simulink subsystem "PvtSubSys_DMS"  (R2020b)
settings: Solver=VariableStepAuto  StartTime=0.0  StopTime=10.0  RelTol=1e-3
undefined symbols (not defined in the file): DMS5, DS, P_DMS_tDSGoodUnbeliv2LowDistrctn, P_DMS_tDSGoodUnbeliv2LowDrowsns, P_DMS_tDSGoodUnbeliv2MidDistractn, P_DMS_tDSGoodUnbeliv2MidDrowsns, P_DMS_tDSLow2MidDistractn, P_DMS_tDSLow2MidDrowsns, P_DMS_tDSOther2Hi1Distractn, P_DMS_tDSOther2Hi1Drowsns, P_DMS_tDSOther2Hi2Distractn, P_DMS_tDSOther2Hi2Drowsns
libraries: simulink x92, TrueDurationTime x22
(part 1 of 2)
settings Model: Creator=GW00184765  LastModifiedBy=GW00133806

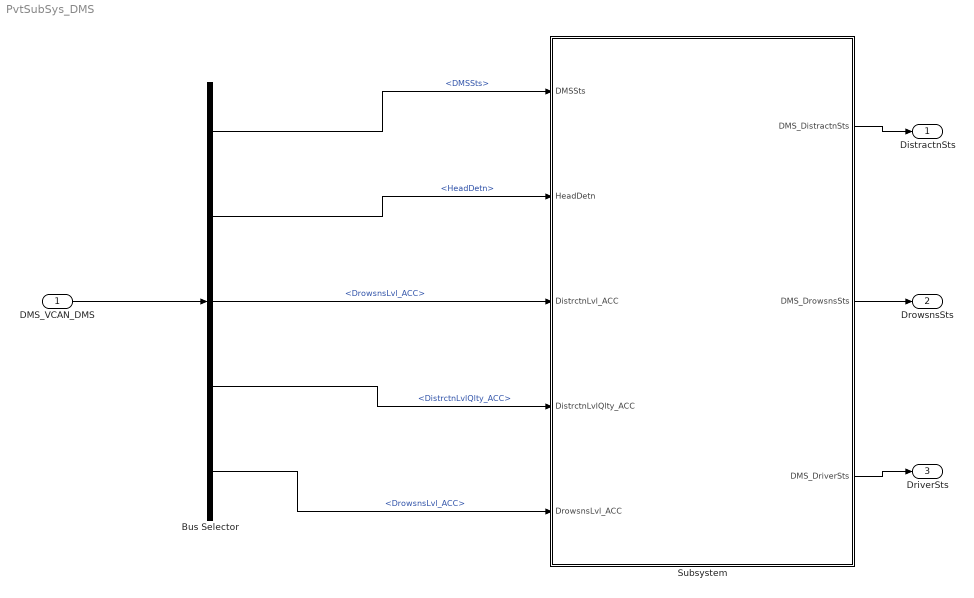
== system PvtSubSys_DMS ==
  DMS_VCAN_DMS : Inport  OutDataTypeStr=Bus: VCAN_DMS_MSG_BUS  PortDimensions=1  BusOutputAsStruct=on
  Bus Selector : BusSelector  OutputSignals=DMSSts,HeadDetn,DrowsnsLvl_ACC,DistrctnLvlQlty_ACC,DrowsnsLvl_ACC
  Subsystem : Subsystem
  DistractnSts : Outport  OutDataTypeStr=uint8  PortDimensions=1  BusOutputAsStruct=on
  DrowsnsSts : Outport  Port=2  OutDataTypeStr=uint8  PortDimensions=1  BusOutputAsStruct=on
  DriverSts : Outport  Port=3  OutDataTypeStr=uint8  PortDimensions=1  BusOutputAsStruct=on
  wires:
  Bus Selector/5 -> Subsystem/5(DrowsnsLvl_ACC)  "<DrowsnsLvl_ACC>"
  Bus Selector/2 -> Subsystem/2(HeadDetn)  "<HeadDetn>"
  Bus Selector/4 -> Subsystem/4(DistrctnLvlQlty_ACC)  "<DistrctnLvlQlty_ACC>"
  DMS_VCAN_DMS/1 -> Bus Selector/1
  Bus Selector/1 -> Subsystem/1(DMSSts)  "<DMSSts>"
  Bus Selector/3 -> Subsystem/3(DistrctnLvl_ACC)  "<DrowsnsLvl_ACC>"
  Subsystem/2(DMS_DrowsnsSts) -> DrowsnsSts/1
  Subsystem/1(DMS_DistractnSts) -> DistractnSts/1
  Subsystem/3(DMS_DriverSts) -> DriverSts/1

== system PvtSubSys_DMS/Subsystem ==
  DMSSts : Inport  OutDataTypeStr=uint8  PortDimensions=1  Interpolate=off  BusOutputAsStruct=on
  HeadDetn : Inport  Port=2  OutDataTypeStr=boolean  PortDimensions=1  Interpolate=off  BusOutputAsStruct=on
  DistrctnLvl_ACC : Inport  Port=3  OutDataTypeStr=uint8  PortDimensions=1  Interpolate=off  BusOutputAsStruct=on
  DistrctnLvlQlty_ACC : Inport  Port=4  OutDataTypeStr=uint8  PortDimensions=1  Interpolate=off  BusOutputAsStruct=on
  DrowsnsLvl_ACC : Inport  Port=5  OutDataTypeStr=uint8  PortDimensions=1  Interpolate=off  BusOutputAsStruct=on
  DS : Subsystem  AncestorBlock=DMS5/DS
  DMS_DistractnSts : Outport
  DMS_DrowsnsSts : Outport  Port=2
  DMS_DriverSts : Outport  Port=3
  wires:
  DrowsnsLvl_ACC/1 -> DS/5(canDrowsnsLevel)
  DistrctnLvlQlty_ACC/1 -> DS/4(canDistrctnQlty)
  DistrctnLvl_ACC/1 -> DS/3(canDistrctnLevel)
  DMSSts/1 -> DS/1(canDMSSts)
  HeadDetn/1 -> DS/2(canHeadDetn)
  DS/3(DriverSts) -> DMS_DriverSts/1  "DMS_DriverSts"
  DS/2(DrowsnsSts) -> DMS_DrowsnsSts/1  "DMS_DrowsnsSts"
  DS/1(DistractnSts) -> DMS_DistractnSts/1  "DMS_DistractnSts"

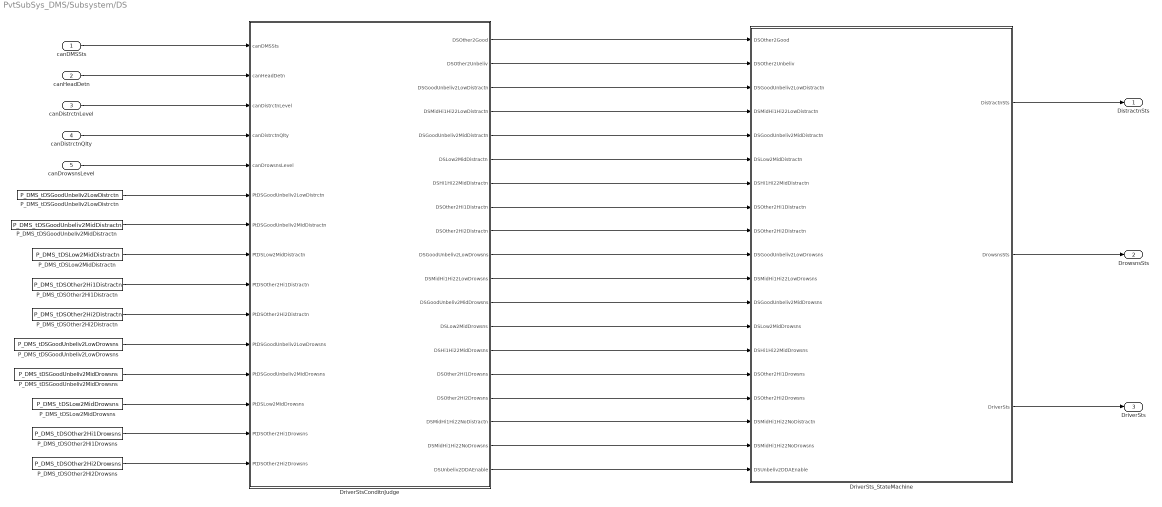
== system PvtSubSys_DMS/Subsystem/DS ==
  canDMSSts : Inport  OutDataTypeStr=uint8
  canHeadDetn : Inport  Port=2  OutDataTypeStr=boolean
  canDistrctnLevel : Inport  Port=3  OutDataTypeStr=uint8
  canDistrctnQlty : Inport  Port=4  OutDataTypeStr=uint8
  canDrowsnsLevel : Inport  Port=5  OutDataTypeStr=uint8
  DriverStsConditnJudge : Subsystem
  DriverSts_StateMachine : Stateflow chart  TreatAsAtomicUnit=on
  P_DMS_tDSGoodUnbeliv2LowDistrctn : Constant  Value=P_DMS_tDSGoodUnbeliv2LowDistrctn
  P_DMS_tDSGoodUnbeliv2LowDrowsns : Constant  Value=P_DMS_tDSGoodUnbeliv2LowDrowsns
  P_DMS_tDSGoodUnbeliv2MidDistractn : Constant  Value=P_DMS_tDSGoodUnbeliv2MidDistractn
  P_DMS_tDSGoodUnbeliv2MidDrowsns : Constant  Value=P_DMS_tDSGoodUnbeliv2MidDrowsns
  P_DMS_tDSLow2MidDistractn : Constant  Value=P_DMS_tDSLow2MidDistractn
  P_DMS_tDSLow2MidDrowsns : Constant  Value=P_DMS_tDSLow2MidDrowsns
  P_DMS_tDSOther2Hi1Distractn : Constant  Value=P_DMS_tDSOther2Hi1Distractn
  P_DMS_tDSOther2Hi1Drowsns : Constant  Value=P_DMS_tDSOther2Hi1Drowsns
  P_DMS_tDSOther2Hi2Distractn : Constant  Value=P_DMS_tDSOther2Hi2Distractn
  P_DMS_tDSOther2Hi2Drowsns : Constant  Value=P_DMS_tDSOther2Hi2Drowsns
  DistractnSts : Outport  OutDataTypeStr=uint8
  DrowsnsSts : Outport  Port=2  OutDataTypeStr=uint8
  DriverSts : Outport  Port=3  OutDataTypeStr=uint8
  wires:
  canDistrctnLevel/1 -> DriverStsConditnJudge/3(canDistrctnLevel)
  canDistrctnQlty/1 -> DriverStsConditnJudge/4(canDistrctnQlty)
  canHeadDetn/1 -> DriverStsConditnJudge/2(canHeadDetn)
  canDrowsnsLevel/1 -> DriverStsConditnJudge/5(canDrowsnsLevel)
  canDMSSts/1 -> DriverStsConditnJudge/1(canDMSSts)
  P_DMS_tDSGoodUnbeliv2LowDistrctn/1 -> DriverStsConditnJudge/6(PtDSGoodUnbeliv2LowDistrctn)
  P_DMS_tDSGoodUnbeliv2MidDistractn/1 -> DriverStsConditnJudge/7(PtDSGoodUnbeliv2MidDistractn)
  P_DMS_tDSLow2MidDistractn/1 -> DriverStsConditnJudge/8(PtDSLow2MidDistractn)
  P_DMS_tDSOther2Hi1Distractn/1 -> DriverStsConditnJudge/9(PtDSOther2Hi1Distractn)
  P_DMS_tDSOther2Hi2Distractn/1 -> DriverStsConditnJudge/10(PtDSOther2Hi2Distractn)
  P_DMS_tDSGoodUnbeliv2LowDrowsns/1 -> DriverStsConditnJudge/11(PtDSGoodUnbeliv2LowDrowsns)
  P_DMS_tDSGoodUnbeliv2MidDrowsns/1 -> DriverStsConditnJudge/12(PtDSGoodUnbeliv2MidDrowsns)
  P_DMS_tDSLow2MidDrowsns/1 -> DriverStsConditnJudge/13(PtDSLow2MidDrowsns)
  P_DMS_tDSOther2Hi1Drowsns/1 -> DriverStsConditnJudge/14(PtDSOther2Hi1Drowsns)
  P_DMS_tDSOther2Hi2Drowsns/1 -> DriverStsConditnJudge/15(PtDSOther2Hi2Drowsns)
  DriverStsConditnJudge/1(DSOther2Good) -> DriverSts_StateMachine/1(DSOther2Good)
  DriverStsConditnJudge/2(DSOther2Unbeliv) -> DriverSts_StateMachine/2(DSOther2Unbeliv)
  DriverStsConditnJudge/3(DSGoodUnbeliv2LowDistractn) -> DriverSts_StateMachine/3(DSGoodUnbeliv2LowDistractn)
  DriverStsConditnJudge/4(DSMidHi1Hi22LowDistractn) -> DriverSts_StateMachine/4(DSMidHi1Hi22LowDistractn)
  DriverStsConditnJudge/5(DSGoodUnbeliv2MidDistractn) -> DriverSts_StateMachine/5(DSGoodUnbeliv2MidDistractn)
  DriverStsConditnJudge/6(DSLow2MidDistractn) -> DriverSts_StateMachine/6(DSLow2MidDistractn)
  DriverStsConditnJudge/7(DSHi1Hi22MidDistractn) -> DriverSts_StateMachine/7(DSHi1Hi22MidDistractn)
  DriverStsConditnJudge/8(DSOther2Hi1Distractn) -> DriverSts_StateMachine/8(DSOther2Hi1Distractn)
  DriverStsConditnJudge/9(DSOther2Hi2Distractn) -> DriverSts_StateMachine/9(DSOther2Hi2Distractn)
  DriverStsConditnJudge/10(DSGoodUnbeliv2LowDrowsns) -> DriverSts_StateMachine/10(DSGoodUnbeliv2LowDrowsns)
  DriverStsConditnJudge/11(DSMidHi1Hi22LowDrowsns) -> DriverSts_StateMachine/11(DSMidHi1Hi22LowDrowsns)
  DriverStsConditnJudge/12(DSGoodUnbeliv2MidDrowsns) -> DriverSts_StateMachine/12(DSGoodUnbeliv2MidDrowsns)
  DriverStsConditnJudge/13(DSLow2MidDrowsns) -> DriverSts_StateMachine/13(DSLow2MidDrowsns)
  DriverStsConditnJudge/14(DSHi1Hi22MidDrowsns) -> DriverSts_StateMachine/14(DSHi1Hi22MidDrowsns)
  DriverStsConditnJudge/15(DSOther2Hi1Drowsns) -> DriverSts_StateMachine/15(DSOther2Hi1Drowsns)
  DriverStsConditnJudge/16(DSOther2Hi2Drowsns) -> DriverSts_StateMachine/16(DSOther2Hi2Drowsns)
  DriverStsConditnJudge/17(DSMidHi1Hi22NoDistractn) -> DriverSts_StateMachine/17(DSMidHi1Hi22NoDistractn)
  DriverStsConditnJudge/18(DSMidHi1Hi22NoDrowsns) -> DriverSts_StateMachine/18(DSMidHi1Hi22NoDrowsns)
  DriverStsConditnJudge/19(DSUnbeliv2DDAEnable) -> DriverSts_StateMachine/19(DSUnbeliv2DDAEnable)
  DriverSts_StateMachine/1(DistractnSts) -> DistractnSts/1
  DriverSts_StateMachine/2(DrowsnsSts) -> DrowsnsSts/1
  DriverSts_StateMachine/3(DriverSts) -> DriverSts/1

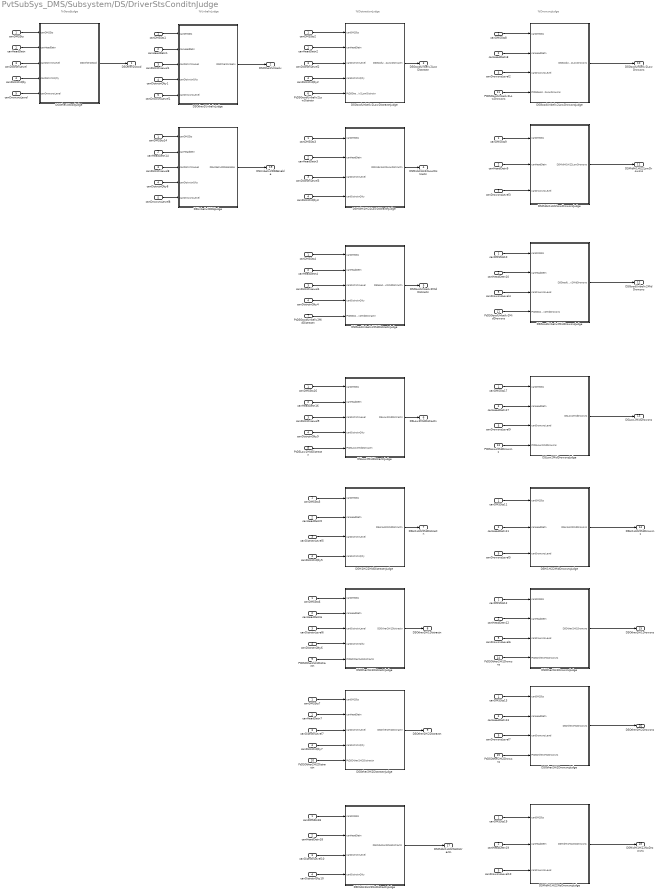
== system PvtSubSys_DMS/Subsystem/DS/DriverStsConditnJudge ==
  note: %GoodJudge
  note: %UnbelivJudge
  note: %DistractionJudge
  note: %DrowsnsJudge
  canDMSSts : Inport
  canHeadDetn : Inport  Port=2
  canDistrctnLevel : Inport  Port=3
  canDistrctnQlty : Inport  Port=4
  canDrowsnsLevel : Inport  Port=5
  PtDSGoodUnbeliv2LowDistrctn : Inport  Port=6
  PtDSGoodUnbeliv2MidDistractn : Inport  Port=7
  PtDSLow2MidDistractn : Inport  Port=8
  PtDSOther2Hi1Distractn : Inport  Port=9
  PtDSOther2Hi2Distractn : Inport  Port=10
  PtDSGoodUnbeliv2LowDrowsns : Inport  Port=11
  PtDSGoodUnbeliv2MidDrowsns : Inport  Port=12
  PtDSLow2MidDrowsns : Inport  Port=13
  PtDSOther2Hi1Drowsns : Inport  Port=14
  PtDSOther2Hi2Drowsns : Inport  Port=15
  DSGoodUnbeliv2LowDistractnJudge : Subsystem
  DSGoodUnbeliv2LowDrowsnsJudge : Subsystem
  DSGoodUnbeliv2MidDistractnJudge : Subsystem
  DSGoodUnbeliv2MidDrowsnsJudge : Subsystem
  DSHi1Hi22MidDistractnJudge : Subsystem
  DSHi1Hi22MidDrowsnsJudge : Subsystem
  DSLow2MidDistractnJudge : Subsystem
  DSLow2MidDrowsnsJudge : Subsystem
  DSMidHi1Hi22LowDistractnJudge : Subsystem
  DSMidHi1Hi22LowDrowsnsJudge : Subsystem
  DSMidHi1Hi22NoDistractnJudge : Subsystem
  DSMidHi1Hi22NoDrowsnsJudge : Subsystem
  DSOther2GoodJudge : Subsystem
  DSOther2Hi1DistractnJudge : Subsystem
  DSOther2Hi1DrowsnsJudge : Subsystem
  DSOther2Hi2DistractnJudge : Subsystem
  DSOther2Hi2DrowsnsJudge : Subsystem
  DSOther2UnbelivJudge : Subsystem
  DSUnbeliv2DDAJudge : Subsystem
  canDMSSts{1..14,16..19} (18 alike) : InportShadow
  canDistrctnLevel{1..10} (10 alike) : InportShadow  Port=3
  canDistrctnQlty{1..10} (10 alike) : InportShadow  Port=4
  canDrowsnsLevel{1..10} (10 alike) : InportShadow  Port=5
  canHeadDetn{1..14,16..19} (18 alike) : InportShadow  Port=2
  DSOther2Good : Outport
  DSOther2Unbeliv : Outport  Port=2
  DSGoodUnbeliv2LowDistractn : Outport  Port=3
  DSMidHi1Hi22LowDistractn : Outport  Port=4
  DSGoodUnbeliv2MidDistractn : Outport  Port=5
  DSLow2MidDistractn : Outport  Port=6
  DSHi1Hi22MidDistractn : Outport  Port=7
  DSOther2Hi1Distractn : Outport  Port=8
  DSOther2Hi2Distractn : Outport  Port=9
  DSGoodUnbeliv2LowDrowsns : Outport  Port=10
  DSMidHi1Hi22LowDrowsns : Outport  Port=11
  DSGoodUnbeliv2MidDrowsns : Outport  Port=12
  DSLow2MidDrowsns : Outport  Port=13
  DSHi1Hi22MidDrowsns : Outport  Port=14
  DSOther2Hi1Drowsns : Outport  Port=15
  DSOther2Hi2Drowsns : Outport  Port=16
  DSMidHi1Hi22NoDistractn : Outport  Port=17
  DSMidHi1Hi22NoDrowsns : Outport  Port=18
  DSUnbeliv2DDAEnable : Outport  Port=19
  wires:
  canDMSSts/1 -> DSOther2GoodJudge/1(canDMSSts)
  DSOther2GoodJudge/1(DSOther2Good) -> DSOther2Good/1
  canHeadDetn/1 -> DSOther2GoodJudge/2(canHeadDetn)
  canDistrctnLevel/1 -> DSOther2GoodJudge/3(canDistrctnLevel)
  canDistrctnQlty/1 -> DSOther2GoodJudge/4(canDistrctnQlty)
  canDrowsnsLevel/1 -> DSOther2GoodJudge/5(canDrowsnsLevel)
  canDMSSts1/1 -> DSOther2UnbelivJudge/1(canDMSSts)
  canHeadDetn1/1 -> DSOther2UnbelivJudge/2(canHeadDetn)
  canDistrctnLevel1/1 -> DSOther2UnbelivJudge/3(canDistrctnLevel)
  canDistrctnQlty1/1 -> DSOther2UnbelivJudge/4(canDistrctnQlty)
  canDrowsnsLevel1/1 -> DSOther2UnbelivJudge/5(canDrowsnsLevel)
  DSOther2UnbelivJudge/1(DSOther2Unbeliv) -> DSOther2Unbeliv/1
  DSGoodUnbeliv2LowDistractnJudge/1(DSGoodUnbeliv2LowDistractn) -> DSGoodUnbeliv2LowDistractn/1
  canDMSSts2/1 -> DSGoodUnbeliv2LowDistractnJudge/1(canDMSSts)
  canHeadDetn2/1 -> DSGoodUnbeliv2LowDistractnJudge/2(canHeadDetn)
  canDistrctnLevel2/1 -> DSGoodUnbeliv2LowDistractnJudge/3(canDistrctnLevel)
  canDistrctnQlty2/1 -> DSGoodUnbeliv2LowDistractnJudge/4(canDistrctnQlty)
  canDMSSts3/1 -> DSMidHi1Hi22LowDistractnJudge/1(canDMSSts)
  canHeadDetn3/1 -> DSMidHi1Hi22LowDistractnJudge/2(canHeadDetn)
  canDistrctnLevel3/1 -> DSMidHi1Hi22LowDistractnJudge/3(canDistrctnLevel)
  canDistrctnQlty3/1 -> DSMidHi1Hi22LowDistractnJudge/4(canDistrctnQlty)
  DSMidHi1Hi22LowDistractnJudge/1(DSMidHi1Hi22LowDistractn) -> DSMidHi1Hi22LowDistractn/1
  canDMSSts4/1 -> DSGoodUnbeliv2MidDistractnJudge/1(canDMSSts)
  canHeadDetn4/1 -> DSGoodUnbeliv2MidDistractnJudge/2(canHeadDetn)
  canDistrctnLevel4/1 -> DSGoodUnbeliv2MidDistractnJudge/3(canDistrctnLevel)
  canDistrctnQlty4/1 -> DSGoodUnbeliv2MidDistractnJudge/4(canDistrctnQlty)
  DSGoodUnbeliv2MidDistractnJudge/1(DSGoodUnbeliv2MidDistractn) -> DSGoodUnbeliv2MidDistractn/1
  canDMSSts5/1 -> DSHi1Hi22MidDistractnJudge/1(canDMSSts)
  canHeadDetn5/1 -> DSHi1Hi22MidDistractnJudge/2(canHeadDetn)
  canDistrctnLevel5/1 -> DSHi1Hi22MidDistractnJudge/3(canDistrctnLevel)
  canDistrctnQlty5/1 -> DSHi1Hi22MidDistractnJudge/4(canDistrctnQlty)
  DSHi1Hi22MidDistractnJudge/1(DSHi1Hi22MidDistractn) -> DSHi1Hi22MidDistractn/1
  DSOther2Hi1DistractnJudge/1(DSOther2Hi1Distractn) -> DSOther2Hi1Distractn/1
  canDMSSts6/1 -> DSOther2Hi1DistractnJudge/1(canDMSSts)
  canHeadDetn6/1 -> DSOther2Hi1DistractnJudge/2(canHeadDetn)
  canDistrctnLevel6/1 -> DSOther2Hi1DistractnJudge/3(canDistrctnLevel)
  canDistrctnQlty6/1 -> DSOther2Hi1DistractnJudge/4(canDistrctnQlty)
  DSOther2Hi2DistractnJudge/1(DSOther2Hi2Distractn) -> DSOther2Hi2Distractn/1
  canDMSSts7/1 -> DSOther2Hi2DistractnJudge/1(canDMSSts)
  canHeadDetn7/1 -> DSOther2Hi2DistractnJudge/2(canHeadDetn)
  canDistrctnLevel7/1 -> DSOther2Hi2DistractnJudge/3(canDistrctnLevel)
  canDistrctnQlty7/1 -> DSOther2Hi2DistractnJudge/4(canDistrctnQlty)
  DSGoodUnbeliv2LowDrowsnsJudge/1(DSGoodUnbeliv2LowDrowsns) -> DSGoodUnbeliv2LowDrowsns/1
  canDMSSts8/1 -> DSGoodUnbeliv2LowDrowsnsJudge/1(canDMSSts)
  canHeadDetn8/1 -> DSGoodUnbeliv2LowDrowsnsJudge/2(canHeadDetn)
  canDrowsnsLevel2/1 -> DSGoodUnbeliv2LowDrowsnsJudge/3(canDrowsnsLevel)
  DSMidHi1Hi22LowDrowsnsJudge/1(DSMidHi1Hi22LowDrowsns) -> DSMidHi1Hi22LowDrowsns/1
  canDMSSts9/1 -> DSMidHi1Hi22LowDrowsnsJudge/1(canDMSSts)
  canHeadDetn9/1 -> DSMidHi1Hi22LowDrowsnsJudge/2(canHeadDetn)
  canDrowsnsLevel3/1 -> DSMidHi1Hi22LowDrowsnsJudge/3(canDrowsnsLevel)
  canDMSSts10/1 -> DSGoodUnbeliv2MidDrowsnsJudge/1(canDMSSts)
  canHeadDetn10/1 -> DSGoodUnbeliv2MidDrowsnsJudge/2(canHeadDetn)
  canDrowsnsLevel4/1 -> DSGoodUnbeliv2MidDrowsnsJudge/3(canDrowsnsLevel)
  DSGoodUnbeliv2MidDrowsnsJudge/1(DSGoodUnbeliv2MidDrowsns) -> DSGoodUnbeliv2MidDrowsns/1
  DSHi1Hi22MidDrowsnsJudge/1(DSHi1Hi22MidDrowsns) -> DSHi1Hi22MidDrowsns/1
  canDrowsnsLevel5/1 -> DSHi1Hi22MidDrowsnsJudge/3(canDrowsnsLevel)
  canHeadDetn11/1 -> DSHi1Hi22MidDrowsnsJudge/2(canHeadDetn)
  canDMSSts11/1 -> DSHi1Hi22MidDrowsnsJudge/1(canDMSSts)
  canDMSSts12/1 -> DSOther2Hi1DrowsnsJudge/1(canDMSSts)
  canHeadDetn12/1 -> DSOther2Hi1DrowsnsJudge/2(canHeadDetn)
  canDrowsnsLevel6/1 -> DSOther2Hi1DrowsnsJudge/3(canDrowsnsLevel)
  DSOther2Hi1DrowsnsJudge/1(DSOther2Hi1Drowsns) -> DSOther2Hi1Drowsns/1
  canDrowsnsLevel7/1 -> DSOther2Hi2DrowsnsJudge/3(canDrowsnsLevel)
  canHeadDetn13/1 -> DSOther2Hi2DrowsnsJudge/2(canHeadDetn)
  canDMSSts13/1 -> DSOther2Hi2DrowsnsJudge/1(canDMSSts)
  DSOther2Hi2DrowsnsJudge/1(DSOther2Hi2Drowsns) -> DSOther2Hi2Drowsns/1
  DSLow2MidDistractnJudge/1(DSLow2MidDistractn) -> DSLow2MidDistractn/1
  canDistrctnQlty9/1 -> DSLow2MidDistractnJudge/4(canDistrctnQlty)
  canDistrctnLevel9/1 -> DSLow2MidDistractnJudge/3(canDistrctnLevel)
  canHeadDetn16/1 -> DSLow2MidDistractnJudge/2(canHeadDetn)
  canDMSSts16/1 -> DSLow2MidDistractnJudge/1(canDMSSts)
  canDrowsnsLevel9/1 -> DSLow2MidDrowsnsJudge/3(canDrowsnsLevel)
  canHeadDetn17/1 -> DSLow2MidDrowsnsJudge/2(canHeadDetn)
  canDMSSts17/1 -> DSLow2MidDrowsnsJudge/1(canDMSSts)
  DSLow2MidDrowsnsJudge/1(DSLow2MidDrowsns) -> DSLow2MidDrowsns/1
  canDistrctnQlty10/1 -> DSMidHi1Hi22NoDistractnJudge/4(canDistrctnQlty)
  canDistrctnLevel10/1 -> DSMidHi1Hi22NoDistractnJudge/3(canDistrctnLevel)
  canHeadDetn18/1 -> DSMidHi1Hi22NoDistractnJudge/2(canHeadDetn)
  canDMSSts18/1 -> DSMidHi1Hi22NoDistractnJudge/1(canDMSSts)
  DSMidHi1Hi22NoDistractnJudge/1(DSMidHi1Hi22NoDistractn) -> DSMidHi1Hi22NoDistractn/1
  canDrowsnsLevel10/1 -> DSMidHi1Hi22NoDrowsnsJudge/3(canDrowsnsLevel)
  canHeadDetn19/1 -> DSMidHi1Hi22NoDrowsnsJudge/2(canHeadDetn)
  canDMSSts19/1 -> DSMidHi1Hi22NoDrowsnsJudge/1(canDMSSts)
  DSMidHi1Hi22NoDrowsnsJudge/1(DSMidHi1Hi22NoDrowsns) -> DSMidHi1Hi22NoDrowsns/1
  canDrowsnsLevel8/1 -> DSUnbeliv2DDAJudge/5(canDrowsnsLevel)
  canDistrctnQlty8/1 -> DSUnbeliv2DDAJudge/4(canDistrctnQlty)
  canDistrctnLevel8/1 -> DSUnbeliv2DDAJudge/3(canDistrctnLevel)
  canHeadDetn14/1 -> DSUnbeliv2DDAJudge/2(canHeadDetn)
  canDMSSts14/1 -> DSUnbeliv2DDAJudge/1(canDMSSts)
  DSUnbeliv2DDAJudge/1(DSUnbeliv2DDAEnable) -> DSUnbeliv2DDAEnable/1
  PtDSGoodUnbeliv2LowDistrctn/1 -> DSGoodUnbeliv2LowDistractnJudge/5(PtDSGoodUnbeliv2LowDistrctn)
  PtDSGoodUnbeliv2MidDistractn/1 -> DSGoodUnbeliv2MidDistractnJudge/5(PtDSGoodUnbeliv2MidDistractn)
  PtDSLow2MidDistractn/1 -> DSLow2MidDistractnJudge/5(PtDSLow2MidDistractn)
  PtDSOther2Hi1Distractn/1 -> DSOther2Hi1DistractnJudge/5(PtDSOther2Hi1Distractn)
  PtDSOther2Hi2Distractn/1 -> DSOther2Hi2DistractnJudge/5(PtDSOther2Hi2Distractn)
  PtDSGoodUnbeliv2LowDrowsns/1 -> DSGoodUnbeliv2LowDrowsnsJudge/4(PtDSGoodUnbeliv2LowDrowsns)
  PtDSGoodUnbeliv2MidDrowsns/1 -> DSGoodUnbeliv2MidDrowsnsJudge/4(PtDSGoodUnbeliv2MidDrowsns)
  PtDSLow2MidDrowsns/1 -> DSLow2MidDrowsnsJudge/4(PtDSLow2MidDrowsns)
  PtDSOther2Hi1Drowsns/1 -> DSOther2Hi1DrowsnsJudge/4(PtDSOther2Hi1Drowsns)
  PtDSOther2Hi2Drowsns/1 -> DSOther2Hi2DrowsnsJudge/4(PtDSOther2Hi2Drowsns)

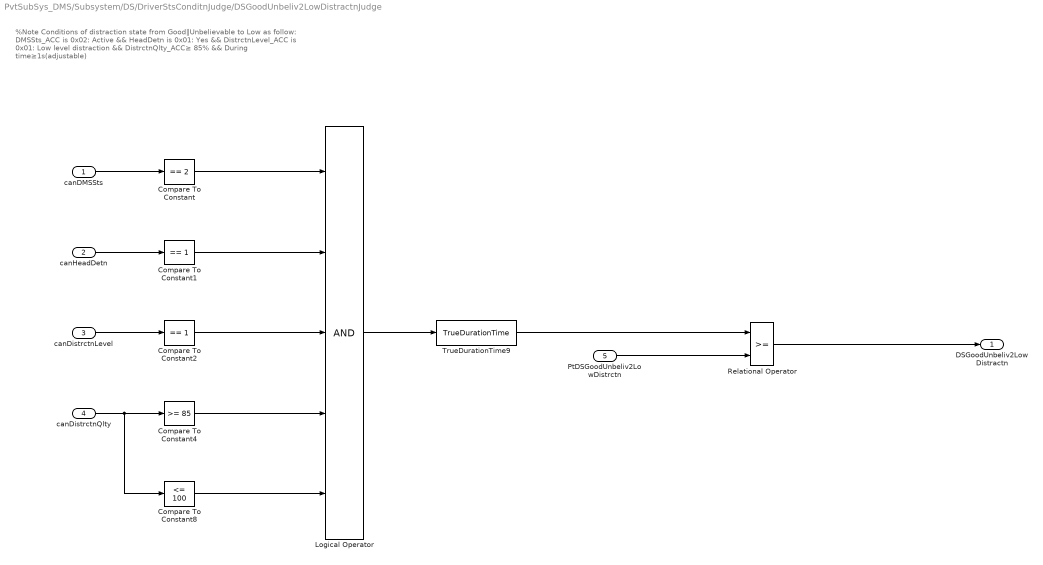
== system PvtSubSys_DMS/Subsystem/DS/DriverStsConditnJudge/DSGoodUnbeliv2LowDistractnJudge ==
  note: %Note
      | Conditions of distraction state from Good∥Unbelievable to Low as follow:
      | DMSSts_ACC is 0x02: Active
      | && HeadDetn is 0x01: Yes
      | && DistrctnLevel_ACC is 0x01: Low level distraction
      | && DistrctnQlty_ACC≥ 85%
      | && During time≥1s(adjustable)
  canDMSSts : Inport
  canHeadDetn : Inport  Port=2
  canDistrctnLevel : Inport  Port=3
  canDistrctnQlty : Inport  Port=4
  PtDSGoodUnbeliv2LowDistrctn : Inport  Port=5
  Compare To Constant : simulink/Logic and Bit Operations/Compare To Constant  relop===  const=2  OutDataTypeStr=boolean
  Compare To Constant1 : simulink/Logic and Bit Operations/Compare To Constant  relop===  const=1  OutDataTypeStr=boolean
  Compare To Constant2 : simulink/Logic and Bit Operations/Compare To Constant  relop===  const=1  OutDataTypeStr=boolean
  Compare To Constant4 : simulink/Logic and Bit Operations/Compare To Constant  relop=>=  const=85  OutDataTypeStr=boolean
  Compare To Constant8 : simulink/Logic and Bit Operations/Compare To Constant  relop=<=  const=100  OutDataTypeStr=boolean
  Logical Operator : Logic  Inputs=5  AllPortsSameDT=off  OutDataTypeStr=boolean
  Relational Operator : RelationalOperator  OutDataTypeStr=boolean  RndMeth=Simplest
  TrueDurationTime9 : TrueDurationTime/TrueDurationTime  TCycle=0.02
  DSGoodUnbeliv2LowDistractn : Outport
  wires:
  canDMSSts/1 -> Compare To Constant/1
  canHeadDetn/1 -> Compare To Constant1/1
  canDistrctnLevel/1 -> Compare To Constant2/1
  Logical Operator/1 -> TrueDurationTime9/1
  TrueDurationTime9/1 -> Relational Operator/1
  canDistrctnQlty/1 -> Compare To Constant8/1, Compare To Constant4/1
  Compare To Constant1/1 -> Logical Operator/2
  Compare To Constant/1 -> Logical Operator/1
  Compare To Constant2/1 -> Logical Operator/3
  Compare To Constant4/1 -> Logical Operator/4
  Compare To Constant8/1 -> Logical Operator/5
  Relational Operator/1 -> DSGoodUnbeliv2LowDistractn/1
  PtDSGoodUnbeliv2LowDistrctn/1 -> Relational Operator/2

== system PvtSubSys_DMS/Subsystem/DS/DriverStsConditnJudge/DSGoodUnbeliv2LowDrowsnsJudge ==
  note: %Note
      | Conditions of drowsns state from Good∥Unbelievable to Low as follow:
      | DMSSts_ACC is 0x02: Active
      | && HeadDetn is 0x01: Yes
      | && DrowsnsLevel_ACC is 0x1: Low level Drowsiness
      | && DrowsnsQlty_ACC≥85%
      | && During time≥3s(adjustable)
  canDMSSts : Inport
  canHeadDetn : Inport  Port=2
  canDrowsnsLevel : Inport  Port=3
  PtDSGoodUnbeliv2LowDrowsns : Inport  Port=4
  Compare To Constant : simulink/Logic and Bit Operations/Compare To Constant  relop===  const=2  OutDataTypeStr=boolean
  Compare To Constant1 : simulink/Logic and Bit Operations/Compare To Constant  relop===  const=1  OutDataTypeStr=boolean
  Compare To Constant2 : simulink/Logic and Bit Operations/Compare To Constant  relop===  const=1  OutDataTypeStr=boolean
  Logical Operator : Logic  Inputs=3  AllPortsSameDT=off  OutDataTypeStr=boolean
  Relational Operator : RelationalOperator  OutDataTypeStr=boolean  RndMeth=Simplest
  TrueDurationTime9 : TrueDurationTime/TrueDurationTime  TCycle=0.02
  DSGoodUnbeliv2LowDrowsns : Outport
  wires:
  Relational Operator/1 -> DSGoodUnbeliv2LowDrowsns/1
  Compare To Constant2/1 -> Logical Operator/3
  Compare To Constant/1 -> Logical Operator/1
  Compare To Constant1/1 -> Logical Operator/2
  TrueDurationTime9/1 -> Relational Operator/1
  Logical Operator/1 -> TrueDurationTime9/1
  canDrowsnsLevel/1 -> Compare To Constant2/1
  canHeadDetn/1 -> Compare To Constant1/1
  canDMSSts/1 -> Compare To Constant/1
  PtDSGoodUnbeliv2LowDrowsns/1 -> Relational Operator/2

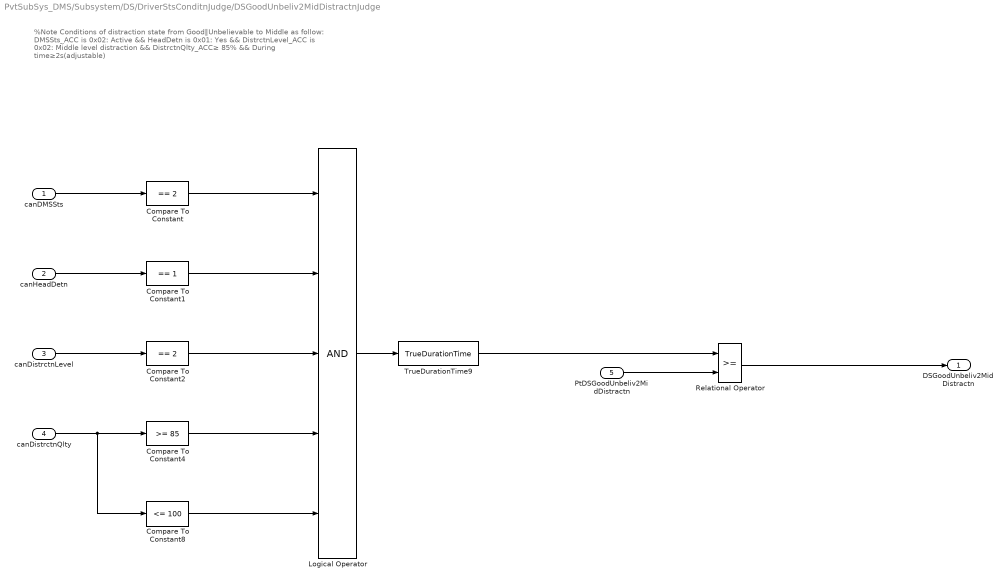
== system PvtSubSys_DMS/Subsystem/DS/DriverStsConditnJudge/DSGoodUnbeliv2MidDistractnJudge ==
  note: %Note
      | Conditions of distraction state from Good∥Unbelievable to Middle as follow:
      | DMSSts_ACC is 0x02: Active
      | && HeadDetn is 0x01: Yes
      | && DistrctnLevel_ACC is 0x02: Middle level distraction
      | && DistrctnQlty_ACC≥ 85%
      | && During time≥2s(adjustable)
  canDMSSts : Inport
  canHeadDetn : Inport  Port=2
  canDistrctnLevel : Inport  Port=3
  canDistrctnQlty : Inport  Port=4
  PtDSGoodUnbeliv2MidDistractn : Inport  Port=5
  Compare To Constant : simulink/Logic and Bit Operations/Compare To Constant  relop===  const=2  OutDataTypeStr=boolean
  Compare To Constant1 : simulink/Logic and Bit Operations/Compare To Constant  relop===  const=1  OutDataTypeStr=boolean
  Compare To Constant2 : simulink/Logic and Bit Operations/Compare To Constant  relop===  const=2  OutDataTypeStr=boolean
  Compare To Constant4 : simulink/Logic and Bit Operations/Compare To Constant  relop=>=  const=85  OutDataTypeStr=boolean
  Compare To Constant8 : simulink/Logic and Bit Operations/Compare To Constant  relop=<=  const=100  OutDataTypeStr=boolean
  Logical Operator : Logic  Inputs=5  AllPortsSameDT=off  OutDataTypeStr=boolean
  Relational Operator : RelationalOperator  OutDataTypeStr=boolean  RndMeth=Simplest
  TrueDurationTime9 : TrueDurationTime/TrueDurationTime  TCycle=0.02
  DSGoodUnbeliv2MidDistractn : Outport
  wires:
  canDMSSts/1 -> Compare To Constant/1
  canHeadDetn/1 -> Compare To Constant1/1
  canDistrctnLevel/1 -> Compare To Constant2/1
  Logical Operator/1 -> TrueDurationTime9/1
  canDistrctnQlty/1 -> Compare To Constant8/1, Compare To Constant4/1
  Compare To Constant1/1 -> Logical Operator/2
  Compare To Constant/1 -> Logical Operator/1
  Compare To Constant2/1 -> Logical Operator/3
  Compare To Constant4/1 -> Logical Operator/4
  Compare To Constant8/1 -> Logical Operator/5
  Relational Operator/1 -> DSGoodUnbeliv2MidDistractn/1
  PtDSGoodUnbeliv2MidDistractn/1 -> Relational Operator/2
  TrueDurationTime9/1 -> Relational Operator/1

== system PvtSubSys_DMS/Subsystem/DS/DriverStsConditnJudge/DSGoodUnbeliv2MidDrowsnsJudge ==
  note: %Note
      | Conditions of drowsns state from Good∥Unbelievable to Middle as follow:
      | DMSSts_ACC is 0x02: Active
      | && HeadDetn is 0x01: Yes
      | && DrowsnsLevel_ACC is 0x2: Middle level Drowsiness
      | && DrowsnsQlty_ACC≥85%
      | && During time≥3s(adjustable)
  canDMSSts : Inport
  canHeadDetn : Inport  Port=2
  canDrowsnsLevel : Inport  Port=3
  PtDSGoodUnbeliv2MidDrowsns : Inport  Port=4
  Compare To Constant : simulink/Logic and Bit Operations/Compare To Constant  relop===  const=2  OutDataTypeStr=boolean
  Compare To Constant1 : simulink/Logic and Bit Operations/Compare To Constant  relop===  const=1  OutDataTypeStr=boolean
  Compare To Constant2 : simulink/Logic and Bit Operations/Compare To Constant  relop===  const=2  OutDataTypeStr=boolean
  Logical Operator : Logic  Inputs=3  AllPortsSameDT=off  OutDataTypeStr=boolean
  Relational Operator : RelationalOperator  OutDataTypeStr=boolean  RndMeth=Simplest
  TrueDurationTime9 : TrueDurationTime/TrueDurationTime  TCycle=0.02
  DSGoodUnbeliv2MidDrowsns : Outport
  wires:
  Compare To Constant2/1 -> Logical Operator/3
  Compare To Constant/1 -> Logical Operator/1
  Compare To Constant1/1 -> Logical Operator/2
  Relational Operator/1 -> DSGoodUnbeliv2MidDrowsns/1
  TrueDurationTime9/1 -> Relational Operator/1
  Logical Operator/1 -> TrueDurationTime9/1
  canDrowsnsLevel/1 -> Compare To Constant2/1
  canHeadDetn/1 -> Compare To Constant1/1
  canDMSSts/1 -> Compare To Constant/1
  PtDSGoodUnbeliv2MidDrowsns/1 -> Relational Operator/2

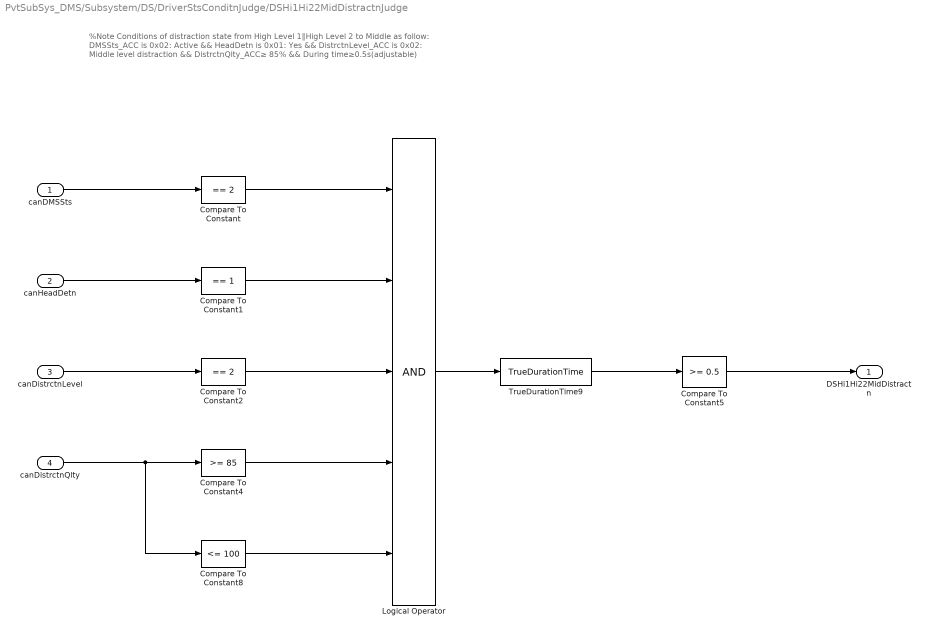
== system PvtSubSys_DMS/Subsystem/DS/DriverStsConditnJudge/DSHi1Hi22MidDistractnJudge ==
  note: %Note
      | Conditions of distraction state from High Level 1∥High Level 2 to Middle as follow:
      | DMSSts_ACC is 0x02: Active
      | && HeadDetn is 0x01: Yes
      | && DistrctnLevel_ACC is 0x02: Middle level distraction
      | && DistrctnQlty_ACC≥ 85%
      | && During time≥0.5s(adjustable)
  canDMSSts : Inport
  canHeadDetn : Inport  Port=2
  canDistrctnLevel : Inport  Port=3
  canDistrctnQlty : Inport  Port=4
  Compare To Constant : simulink/Logic and Bit Operations/Compare To Constant  relop===  const=2  OutDataTypeStr=boolean
  Compare To Constant1 : simulink/Logic and Bit Operations/Compare To Constant  relop===  const=1  OutDataTypeStr=boolean
  Compare To Constant2 : simulink/Logic and Bit Operations/Compare To Constant  relop===  const=2  OutDataTypeStr=boolean
  Compare To Constant4 : simulink/Logic and Bit Operations/Compare To Constant  relop=>=  const=85  OutDataTypeStr=boolean
  Compare To Constant5 : simulink/Logic and Bit Operations/Compare To Constant  relop=>=  const=0.5  OutDataTypeStr=boolean
  Compare To Constant8 : simulink/Logic and Bit Operations/Compare To Constant  relop=<=  const=100  OutDataTypeStr=boolean
  Logical Operator : Logic  Inputs=5  AllPortsSameDT=off  OutDataTypeStr=boolean
  TrueDurationTime9 : TrueDurationTime/TrueDurationTime  TCycle=0.02
  DSHi1Hi22MidDistractn : Outport
  wires:
  Compare To Constant5/1 -> DSHi1Hi22MidDistractn/1
  Compare To Constant8/1 -> Logical Operator/5
  Compare To Constant4/1 -> Logical Operator/4
  Compare To Constant2/1 -> Logical Operator/3
  Compare To Constant/1 -> Logical Operator/1
  Compare To Constant1/1 -> Logical Operator/2
  canDistrctnQlty/1 -> Compare To Constant4/1, Compare To Constant8/1
  TrueDurationTime9/1 -> Compare To Constant5/1
  Logical Operator/1 -> TrueDurationTime9/1
  canDistrctnLevel/1 -> Compare To Constant2/1
  canHeadDetn/1 -> Compare To Constant1/1
  canDMSSts/1 -> Compare To Constant/1

== system PvtSubSys_DMS/Subsystem/DS/DriverStsConditnJudge/DSHi1Hi22MidDrowsnsJudge ==
  note: %Note
      | Conditions of drowsns state from High Level 1∥High Level 2 to Middle as follow:
      | DMSSts_ACC is 0x02: Active
      | && HeadDetn is 0x01: Yes
      | && DrowsnsLevel_ACC is 0x2: Middle level Drowsiness
      | && DrowsnsQlty_ACC≥85%
      | && During time≥0.5s(adjustable)
  canDMSSts : Inport
  canHeadDetn : Inport  Port=2
  canDrowsnsLevel : Inport  Port=3
  Compare To Constant : simulink/Logic and Bit Operations/Compare To Constant  relop===  const=2  OutDataTypeStr=boolean
  Compare To Constant1 : simulink/Logic and Bit Operations/Compare To Constant  relop===  const=1  OutDataTypeStr=boolean
  Compare To Constant2 : simulink/Logic and Bit Operations/Compare To Constant  relop===  const=2  OutDataTypeStr=boolean
  Compare To Constant5 : simulink/Logic and Bit Operations/Compare To Constant  relop=>=  const=0.5  OutDataTypeStr=boolean
  Logical Operator : Logic  Inputs=3  AllPortsSameDT=off  OutDataTypeStr=boolean
  TrueDurationTime9 : TrueDurationTime/TrueDurationTime  TCycle=0.02
  DSHi1Hi22MidDrowsns : Outport
  wires:
  canDMSSts/1 -> Compare To Constant/1
  canHeadDetn/1 -> Compare To Constant1/1
  canDrowsnsLevel/1 -> Compare To Constant2/1
  Logical Operator/1 -> TrueDurationTime9/1
  TrueDurationTime9/1 -> Compare To Constant5/1
  Compare To Constant1/1 -> Logical Operator/2
  Compare To Constant/1 -> Logical Operator/1
  Compare To Constant2/1 -> Logical Operator/3
  Compare To Constant5/1 -> DSHi1Hi22MidDrowsns/1

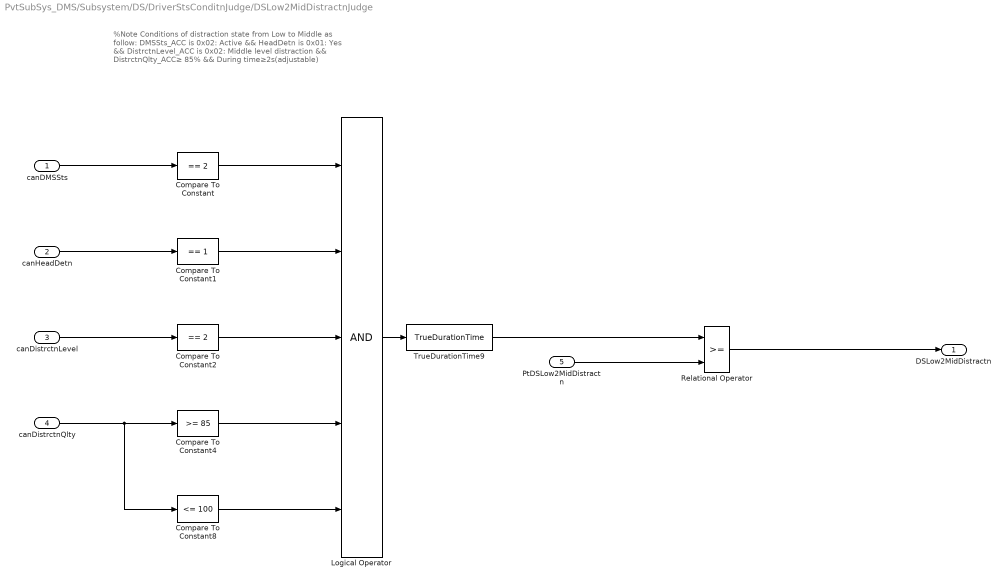
== system PvtSubSys_DMS/Subsystem/DS/DriverStsConditnJudge/DSLow2MidDistractnJudge ==
  note: %Note
      | Conditions of distraction state from Low to Middle as follow:
      | DMSSts_ACC is 0x02: Active
      | && HeadDetn is 0x01: Yes
      | && DistrctnLevel_ACC is 0x02: Middle level distraction
      | && DistrctnQlty_ACC≥ 85%
      | && During time≥2s(adjustable)
  canDMSSts : Inport
  canHeadDetn : Inport  Port=2
  canDistrctnLevel : Inport  Port=3
  canDistrctnQlty : Inport  Port=4
  PtDSLow2MidDistractn : Inport  Port=5
  Compare To Constant : simulink/Logic and Bit Operations/Compare To Constant  relop===  const=2  OutDataTypeStr=boolean
  Compare To Constant1 : simulink/Logic and Bit Operations/Compare To Constant  relop===  const=1  OutDataTypeStr=boolean
  Compare To Constant2 : simulink/Logic and Bit Operations/Compare To Constant  relop===  const=2  OutDataTypeStr=boolean
  Compare To Constant4 : simulink/Logic and Bit Operations/Compare To Constant  relop=>=  const=85  OutDataTypeStr=boolean
  Compare To Constant8 : simulink/Logic and Bit Operations/Compare To Constant  relop=<=  const=100  OutDataTypeStr=boolean
  Logical Operator : Logic  Inputs=5  AllPortsSameDT=off  OutDataTypeStr=boolean
  Relational Operator : RelationalOperator  OutDataTypeStr=boolean  RndMeth=Simplest
  TrueDurationTime9 : TrueDurationTime/TrueDurationTime  TCycle=0.02
  DSLow2MidDistractn : Outport
  wires:
  Relational Operator/1 -> DSLow2MidDistractn/1
  Compare To Constant8/1 -> Logical Operator/5
  Compare To Constant4/1 -> Logical Operator/4
  Compare To Constant2/1 -> Logical Operator/3
  Compare To Constant/1 -> Logical Operator/1
  Compare To Constant1/1 -> Logical Operator/2
  canDistrctnQlty/1 -> Compare To Constant4/1, Compare To Constant8/1
  Logical Operator/1 -> TrueDurationTime9/1
  canDistrctnLevel/1 -> Compare To Constant2/1
  canHeadDetn/1 -> Compare To Constant1/1
  canDMSSts/1 -> Compare To Constant/1
  PtDSLow2MidDistractn/1 -> Relational Operator/2
  TrueDurationTime9/1 -> Relational Operator/1

== system PvtSubSys_DMS/Subsystem/DS/DriverStsConditnJudge/DSLow2MidDrowsnsJudge ==
  note: %Note
      | Conditions of drowsns state from Low to Middle as follow:
      | DMSSts_ACC is 0x02: Active
      | && HeadDetn is 0x01: Yes
      | && DrowsnsLevel_ACC is 0x2: Middle level Drowsiness
      | && DrowsnsQlty_ACC≥85%
      | && During time≥3s(adjustable)
  canDMSSts : Inport
  canHeadDetn : Inport  Port=2
  canDrowsnsLevel : Inport  Port=3
  PtDSLow2MidDrowsns : Inport  Port=4
  Compare To Constant : simulink/Logic and Bit Operations/Compare To Constant  relop===  const=2  OutDataTypeStr=boolean
  Compare To Constant1 : simulink/Logic and Bit Operations/Compare To Constant  relop===  const=1  OutDataTypeStr=boolean
  Compare To Constant2 : simulink/Logic and Bit Operations/Compare To Constant  relop===  const=2  OutDataTypeStr=boolean
  Logical Operator : Logic  Inputs=3  AllPortsSameDT=off  OutDataTypeStr=boolean
  Relational Operator : RelationalOperator  OutDataTypeStr=boolean  RndMeth=Simplest
  TrueDurationTime9 : TrueDurationTime/TrueDurationTime  TCycle=0.02
  DSLow2MidDrowsns : Outport
  wires:
  canDMSSts/1 -> Compare To Constant/1
  canHeadDetn/1 -> Compare To Constant1/1
  canDrowsnsLevel/1 -> Compare To Constant2/1
  Logical Operator/1 -> TrueDurationTime9/1
  TrueDurationTime9/1 -> Relational Operator/1
  Compare To Constant1/1 -> Logical Operator/2
  Compare To Constant/1 -> Logical Operator/1
  Compare To Constant2/1 -> Logical Operator/3
  Relational Operator/1 -> DSLow2MidDrowsns/1
  PtDSLow2MidDrowsns/1 -> Relational Operator/2

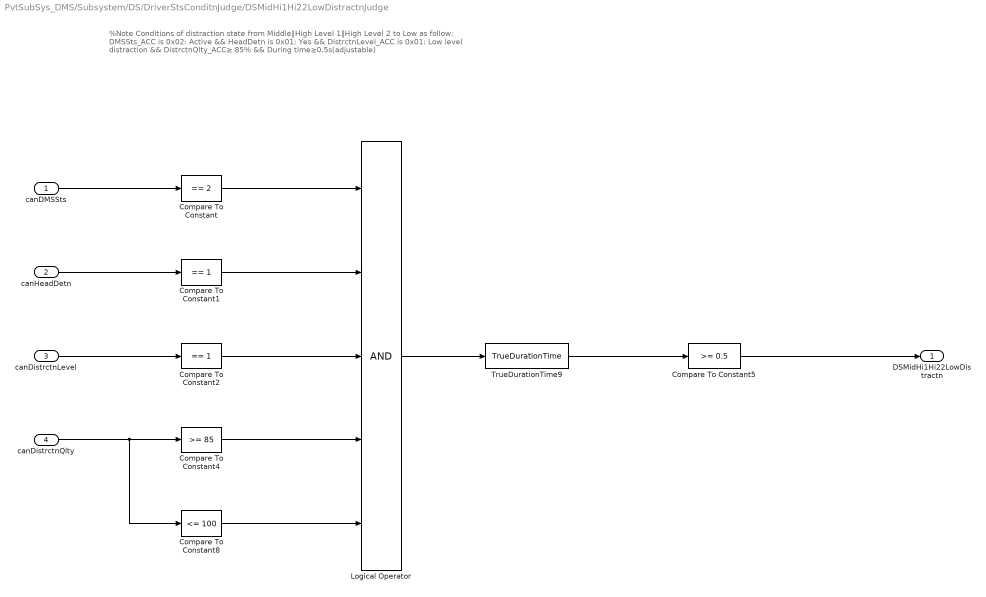
== system PvtSubSys_DMS/Subsystem/DS/DriverStsConditnJudge/DSMidHi1Hi22LowDistractnJudge ==
  note: %Note
      | Conditions of distraction state from Middle∥High Level 1∥High Level 2 to Low as follow:
      | DMSSts_ACC is 0x02: Active
      | && HeadDetn is 0x01: Yes
      | && DistrctnLevel_ACC is 0x01: Low level distraction
      | && DistrctnQlty_ACC≥ 85%
      | && During time≥0.5s(adjustable)
  canDMSSts : Inport
  canHeadDetn : Inport  Port=2
  canDistrctnLevel : Inport  Port=3
  canDistrctnQlty : Inport  Port=4
  Compare To Constant : simulink/Logic and Bit Operations/Compare To Constant  relop===  const=2  OutDataTypeStr=boolean
  Compare To Constant1 : simulink/Logic and Bit Operations/Compare To Constant  relop===  const=1  OutDataTypeStr=boolean
  Compare To Constant2 : simulink/Logic and Bit Operations/Compare To Constant  relop===  const=1  OutDataTypeStr=boolean
  Compare To Constant4 : simulink/Logic and Bit Operations/Compare To Constant  relop=>=  const=85  OutDataTypeStr=boolean
  Compare To Constant5 : simulink/Logic and Bit Operations/Compare To Constant  relop=>=  const=0.5  OutDataTypeStr=boolean
  Compare To Constant8 : simulink/Logic and Bit Operations/Compare To Constant  relop=<=  const=100  OutDataTypeStr=boolean
  Logical Operator : Logic  Inputs=5  AllPortsSameDT=off  OutDataTypeStr=boolean
  TrueDurationTime9 : TrueDurationTime/TrueDurationTime  TCycle=0.02
  DSMidHi1Hi22LowDistractn : Outport
  wires:
  Compare To Constant5/1 -> DSMidHi1Hi22LowDistractn/1
  Compare To Constant8/1 -> Logical Operator/5
  Compare To Constant4/1 -> Logical Operator/4
  Compare To Constant2/1 -> Logical Operator/3
  Compare To Constant/1 -> Logical Operator/1
  Compare To Constant1/1 -> Logical Operator/2
  canDistrctnQlty/1 -> Compare To Constant4/1, Compare To Constant8/1
  Logical Operator/1 -> TrueDurationTime9/1
  canDistrctnLevel/1 -> Compare To Constant2/1
  canHeadDetn/1 -> Compare To Constant1/1
  canDMSSts/1 -> Compare To Constant/1
  TrueDurationTime9/1 -> Compare To Constant5/1

== system PvtSubSys_DMS/Subsystem/DS/DriverStsConditnJudge/DSMidHi1Hi22LowDrowsnsJudge ==
  note: %Note
      | Conditions of drowsns state from Middle∥High Level 1∥High Level 2 to Low as follow:
      | DMSSts_ACC is 0x02: Active
      | && HeadDetn is 0x01: Yes
      | && DrowsnsLevel_ACC is 0x1: Low level Drowsiness
      | && DrowsnsQlty_ACC≥85%
      | && During time≥0.5s(adjustable)
  canDMSSts : Inport
  canHeadDetn : Inport  Port=2
  canDrowsnsLevel : Inport  Port=3
  Compare To Constant : simulink/Logic and Bit Operations/Compare To Constant  relop===  const=2  OutDataTypeStr=boolean
  Compare To Constant1 : simulink/Logic and Bit Operations/Compare To Constant  relop===  const=1  OutDataTypeStr=boolean
  Compare To Constant2 : simulink/Logic and Bit Operations/Compare To Constant  relop===  const=1  OutDataTypeStr=boolean
  Compare To Constant5 : simulink/Logic and Bit Operations/Compare To Constant  relop=>=  const=0.5  OutDataTypeStr=boolean
  Logical Operator : Logic  Inputs=3  AllPortsSameDT=off  OutDataTypeStr=boolean
  TrueDurationTime9 : TrueDurationTime/TrueDurationTime  TCycle=0.02
  DSMidHi1Hi22LowDrowsns : Outport
  wires:
  canDMSSts/1 -> Compare To Constant/1
  canHeadDetn/1 -> Compare To Constant1/1
  canDrowsnsLevel/1 -> Compare To Constant2/1
  Logical Operator/1 -> TrueDurationTime9/1
  Compare To Constant1/1 -> Logical Operator/2
  Compare To Constant/1 -> Logical Operator/1
  Compare To Constant2/1 -> Logical Operator/3
  Compare To Constant5/1 -> DSMidHi1Hi22LowDrowsns/1
  TrueDurationTime9/1 -> Compare To Constant5/1

== system PvtSubSys_DMS/Subsystem/DS/DriverStsConditnJudge/DSMidHi1Hi22NoDistractnJudge ==
  note: %Note
      | In order to cover one case at which distraction is no distraction but drowsns is low/middle/high 1/high2,add this
      | transition from low/middle/high 1/high2 distraction to no distraction.Conditions as follow:
      | DMSSts_ACC is 0x02: Active
      | && HeadDetn is 0x01: Yes
      | && DistrctnLevel_ACC is 0x00: No distraction
      | && DistrctnQlty_ACC≥ 85%
      | && During time is same as time of other to good
  canDMSSts : Inport
  canHeadDetn : Inport  Port=2
  canDistrctnLevel : Inport  Port=3
  canDistrctnQlty : Inport  Port=4
  Compare To Constant : simulink/Logic and Bit Operations/Compare To Constant  relop===  const=2  OutDataTypeStr=boolean
  Compare To Constant1 : simulink/Logic and Bit Operations/Compare To Constant  relop===  const=1  OutDataTypeStr=boolean
  Compare To Constant2 : simulink/Logic and Bit Operations/Compare To Constant  relop===  const=0  OutDataTypeStr=boolean
  Compare To Constant4 : simulink/Logic and Bit Operations/Compare To Constant  relop=>=  const=85  OutDataTypeStr=boolean
  Compare To Constant5 : simulink/Logic and Bit Operations/Compare To Constant  relop=>=  const=0.5  OutDataTypeStr=boolean
  Compare To Constant8 : simulink/Logic and Bit Operations/Compare To Constant  relop=<=  const=100  OutDataTypeStr=boolean
  Logical Operator : Logic  Inputs=5  AllPortsSameDT=off  OutDataTypeStr=boolean
  TrueDurationTime9 : TrueDurationTime/TrueDurationTime  TCycle=0.02
  DSMidHi1Hi22NoDistractn : Outport
  wires:
  Compare To Constant5/1 -> DSMidHi1Hi22NoDistractn/1
  Compare To Constant8/1 -> Logical Operator/5
  Compare To Constant4/1 -> Logical Operator/4
  Compare To Constant2/1 -> Logical Operator/3
  Compare To Constant/1 -> Logical Operator/1
  Compare To Constant1/1 -> Logical Operator/2
  canDistrctnQlty/1 -> Compare To Constant4/1, Compare To Constant8/1
  TrueDurationTime9/1 -> Compare To Constant5/1
  Logical Operator/1 -> TrueDurationTime9/1
  canDistrctnLevel/1 -> Compare To Constant2/1
  canHeadDetn/1 -> Compare To Constant1/1
  canDMSSts/1 -> Compare To Constant/1

== system PvtSubSys_DMS/Subsystem/DS/DriverStsConditnJudge/DSMidHi1Hi22NoDrowsnsJudge ==
  note: %Note
      | In order to cover one case at which drowsns is no drowsiness but distraction is low/middle/high 1/high2,add this
      | transition from low/middle/high 1/high2 drowsiness to no drowsiness.Conditions as follow:
      | DMSSts_ACC is 0x02: Active
      | && HeadDetn is 0x01: Yes
      | && DrowsnsLevel_ACC is：0x0: No Drowsiness
      | && DrowsnsQlty_ACC≥85%
      | && During time is same as time of other to good
  canDMSSts : Inport
  canHeadDetn : Inport  Port=2
  canDrowsnsLevel : Inport  Port=3
  Compare To Constant : simulink/Logic and Bit Operations/Compare To Constant  relop===  const=2  OutDataTypeStr=boolean
  Compare To Constant1 : simulink/Logic and Bit Operations/Compare To Constant  relop===  const=1  OutDataTypeStr=boolean
  Compare To Constant2 : simulink/Logic and Bit Operations/Compare To Constant  relop===  const=0  OutDataTypeStr=boolean
  Compare To Constant5 : simulink/Logic and Bit Operations/Compare To Constant  relop=>=  const=0.5  OutDataTypeStr=boolean
  Logical Operator : Logic  Inputs=3  AllPortsSameDT=off  OutDataTypeStr=boolean
  TrueDurationTime9 : TrueDurationTime/TrueDurationTime  TCycle=0.02
  DSMidHi1Hi22NoDrowsns : Outport
  wires:
  canDMSSts/1 -> Compare To Constant/1
  canHeadDetn/1 -> Compare To Constant1/1
  canDrowsnsLevel/1 -> Compare To Constant2/1
  Logical Operator/1 -> TrueDurationTime9/1
  TrueDurationTime9/1 -> Compare To Constant5/1
  Compare To Constant1/1 -> Logical Operator/2
  Compare To Constant/1 -> Logical Operator/1
  Compare To Constant2/1 -> Logical Operator/3
  Compare To Constant5/1 -> DSMidHi1Hi22NoDrowsns/1

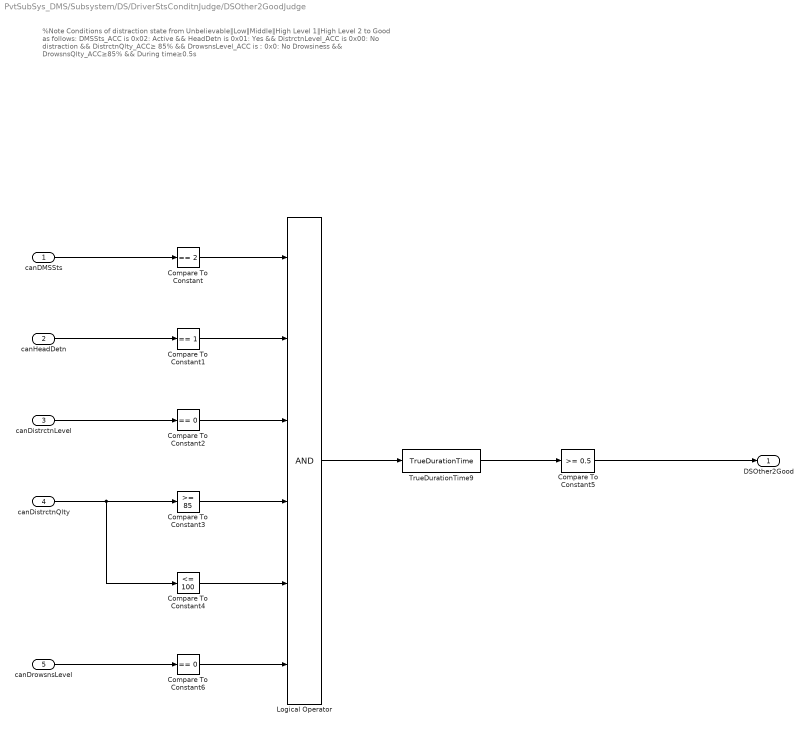
== system PvtSubSys_DMS/Subsystem/DS/DriverStsConditnJudge/DSOther2GoodJudge ==
  note: %Note
      | Conditions of distraction state from Unbelievable∥Low∥Middle∥High Level 1∥High Level 2 to Good as follows:
      | DMSSts_ACC is 0x02: Active
      | && HeadDetn is 0x01: Yes
      | && DistrctnLevel_ACC is 0x00: No distraction
      | && DistrctnQlty_ACC≥ 85%
      | && DrowsnsLevel_ACC is：0x0: No Drowsiness
      | && DrowsnsQlty_ACC≥85%
      | && During time≥0.5s
  canDMSSts : Inport
  canHeadDetn : Inport  Port=2
  canDistrctnLevel : Inport  Port=3
  canDistrctnQlty : Inport  Port=4
  canDrowsnsLevel : Inport  Port=5
  Compare To Constant : simulink/Logic and Bit Operations/Compare To Constant  relop===  const=2  OutDataTypeStr=boolean
  Compare To Constant1 : simulink/Logic and Bit Operations/Compare To Constant  relop===  const=1  OutDataTypeStr=boolean
  Compare To Constant2 : simulink/Logic and Bit Operations/Compare To Constant  relop===  const=0  OutDataTypeStr=boolean
  Compare To Constant3 : simulink/Logic and Bit Operations/Compare To Constant  relop=>=  const=85  OutDataTypeStr=boolean
  Compare To Constant4 : simulink/Logic and Bit Operations/Compare To Constant  relop=<=  const=100  OutDataTypeStr=boolean
  Compare To Constant5 : simulink/Logic and Bit Operations/Compare To Constant  relop=>=  const=0.5  OutDataTypeStr=boolean
  Compare To Constant6 : simulink/Logic and Bit Operations/Compare To Constant  relop===  const=0  OutDataTypeStr=boolean
  Logical Operator : Logic  Inputs=6  AllPortsSameDT=off  OutDataTypeStr=boolean
  TrueDurationTime9 : TrueDurationTime/TrueDurationTime  TCycle=0.02
  DSOther2Good : Outport
  wires:
  canDMSSts/1 -> Compare To Constant/1
  canHeadDetn/1 -> Compare To Constant1/1
  canDistrctnLevel/1 -> Compare To Constant2/1
  canDistrctnQlty/1 -> Compare To Constant4/1, Compare To Constant3/1
  Logical Operator/1 -> TrueDurationTime9/1
  TrueDurationTime9/1 -> Compare To Constant5/1
  canDrowsnsLevel/1 -> Compare To Constant6/1
  Compare To Constant/1 -> Logical Operator/1
  Compare To Constant1/1 -> Logical Operator/2
  Compare To Constant2/1 -> Logical Operator/3
  Compare To Constant3/1 -> Logical Operator/4
  Compare To Constant4/1 -> Logical Operator/5
  Compare To Constant6/1 -> Logical Operator/6
  Compare To Constant5/1 -> DSOther2Good/1

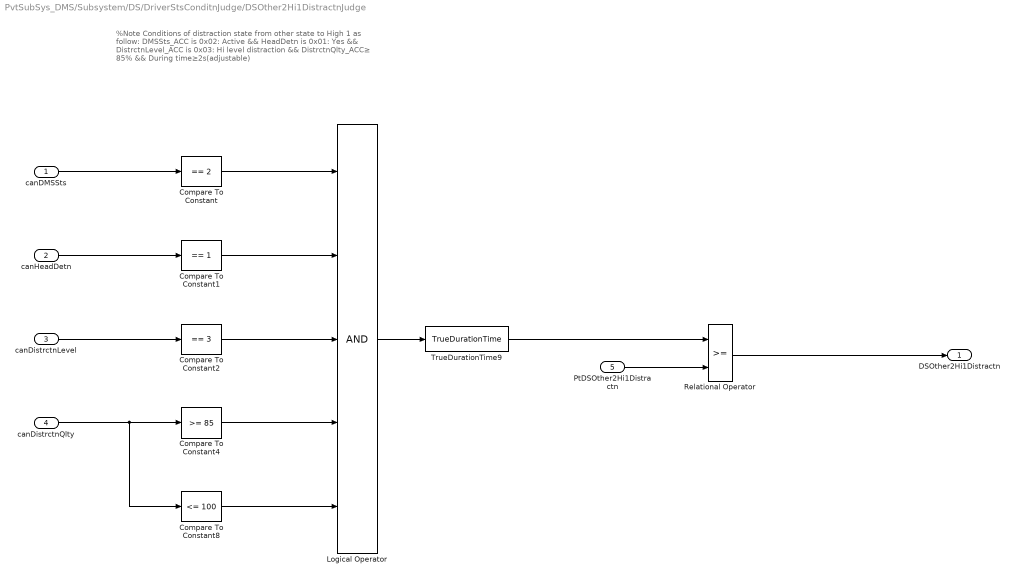
== system PvtSubSys_DMS/Subsystem/DS/DriverStsConditnJudge/DSOther2Hi1DistractnJudge ==
  note: %Note
      | Conditions of distraction state from other state to High 1 as follow:
      | DMSSts_ACC is 0x02: Active
      | && HeadDetn is 0x01: Yes
      | && DistrctnLevel_ACC is 0x03: Hi level distraction
      | && DistrctnQlty_ACC≥ 85%
      | && During time≥2s(adjustable)
  canDMSSts : Inport
  canHeadDetn : Inport  Port=2
  canDistrctnLevel : Inport  Port=3
  canDistrctnQlty : Inport  Port=4
  PtDSOther2Hi1Distractn : Inport  Port=5
  Compare To Constant : simulink/Logic and Bit Operations/Compare To Constant  relop===  const=2  OutDataTypeStr=boolean
  Compare To Constant1 : simulink/Logic and Bit Operations/Compare To Constant  relop===  const=1  OutDataTypeStr=boolean
  Compare To Constant2 : simulink/Logic and Bit Operations/Compare To Constant  relop===  const=3  OutDataTypeStr=boolean
  Compare To Constant4 : simulink/Logic and Bit Operations/Compare To Constant  relop=>=  const=85  OutDataTypeStr=boolean
  Compare To Constant8 : simulink/Logic and Bit Operations/Compare To Constant  relop=<=  const=100  OutDataTypeStr=boolean
  Logical Operator : Logic  Inputs=5  AllPortsSameDT=off  OutDataTypeStr=boolean
  Relational Operator : RelationalOperator  OutDataTypeStr=boolean  RndMeth=Simplest
  TrueDurationTime9 : TrueDurationTime/TrueDurationTime  TCycle=0.02
  DSOther2Hi1Distractn : Outport
  wires:
  Logical Operator/1 -> TrueDurationTime9/1
  canDMSSts/1 -> Compare To Constant/1
  canHeadDetn/1 -> Compare To Constant1/1
  canDistrctnLevel/1 -> Compare To Constant2/1
  canDistrctnQlty/1 -> Compare To Constant8/1, Compare To Constant4/1
  Compare To Constant1/1 -> Logical Operator/2
  Compare To Constant/1 -> Logical Operator/1
  Compare To Constant2/1 -> Logical Operator/3
  Compare To Constant4/1 -> Logical Operator/4
  Compare To Constant8/1 -> Logical Operator/5
  Relational Operator/1 -> DSOther2Hi1Distractn/1
  TrueDurationTime9/1 -> Relational Operator/1
  PtDSOther2Hi1Distractn/1 -> Relational Operator/2

== system PvtSubSys_DMS/Subsystem/DS/DriverStsConditnJudge/DSOther2Hi1DrowsnsJudge ==
  note: %Note
      | Conditions of drowsns state from other state to High 1 as follow:
      | DMSSts_ACC is 0x02: Active
      | && HeadDetn is 0x01: Yes
      | && DrowsnsLevel_ACC is 0x3: Hi level Drowsiness
      | && DrowsnsQlty_ACC≥85%
      | && During time≥0.5s(adjustable)
  canDMSSts : Inport
  canHeadDetn : Inport  Port=2
  canDrowsnsLevel : Inport  Port=3
  PtDSOther2Hi1Drowsns : Inport  Port=4
  Compare To Constant : simulink/Logic and Bit Operations/Compare To Constant  relop===  const=2  OutDataTypeStr=boolean
  Compare To Constant1 : simulink/Logic and Bit Operations/Compare To Constant  relop===  const=1  OutDataTypeStr=boolean
  Compare To Constant2 : simulink/Logic and Bit Operations/Compare To Constant  relop===  const=3  OutDataTypeStr=boolean
  Logical Operator : Logic  Inputs=3  AllPortsSameDT=off  OutDataTypeStr=boolean
  Relational Operator : RelationalOperator  OutDataTypeStr=boolean  RndMeth=Simplest
  TrueDurationTime9 : TrueDurationTime/TrueDurationTime  TCycle=0.02
  DSOther2Hi1Drowsns : Outport
  wires:
  TrueDurationTime9/1 -> Relational Operator/1
  Relational Operator/1 -> DSOther2Hi1Drowsns/1
  Compare To Constant2/1 -> Logical Operator/3
  Compare To Constant/1 -> Logical Operator/1
  Compare To Constant1/1 -> Logical Operator/2
  canDrowsnsLevel/1 -> Compare To Constant2/1
  canHeadDetn/1 -> Compare To Constant1/1
  canDMSSts/1 -> Compare To Constant/1
  Logical Operator/1 -> TrueDurationTime9/1
  PtDSOther2Hi1Drowsns/1 -> Relational Operator/2

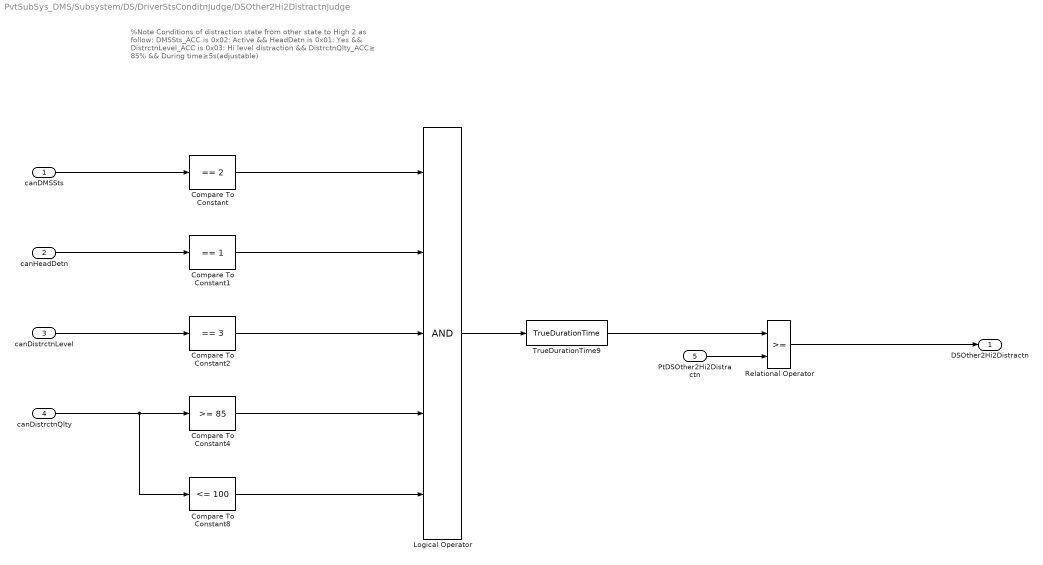
== system PvtSubSys_DMS/Subsystem/DS/DriverStsConditnJudge/DSOther2Hi2DistractnJudge ==
  note: %Note
      | Conditions of distraction state from other state to High 2 as follow:
      | DMSSts_ACC is 0x02: Active
      | && HeadDetn is 0x01: Yes
      | && DistrctnLevel_ACC is 0x03: Hi level distraction
      | && DistrctnQlty_ACC≥ 85%
      | && During time≥5s(adjustable)
  canDMSSts : Inport
  canHeadDetn : Inport  Port=2
  canDistrctnLevel : Inport  Port=3
  canDistrctnQlty : Inport  Port=4
  PtDSOther2Hi2Distractn : Inport  Port=5
  Compare To Constant : simulink/Logic and Bit Operations/Compare To Constant  relop===  const=2  OutDataTypeStr=boolean
  Compare To Constant1 : simulink/Logic and Bit Operations/Compare To Constant  relop===  const=1  OutDataTypeStr=boolean
  Compare To Constant2 : simulink/Logic and Bit Operations/Compare To Constant  relop===  const=3  OutDataTypeStr=boolean
  Compare To Constant4 : simulink/Logic and Bit Operations/Compare To Constant  relop=>=  const=85  OutDataTypeStr=boolean
  Compare To Constant8 : simulink/Logic and Bit Operations/Compare To Constant  relop=<=  const=100  OutDataTypeStr=boolean
  Logical Operator : Logic  Inputs=5  AllPortsSameDT=off  OutDataTypeStr=boolean
  Relational Operator : RelationalOperator  OutDataTypeStr=boolean  RndMeth=Simplest
  TrueDurationTime9 : TrueDurationTime/TrueDurationTime  TCycle=0.02
  DSOther2Hi2Distractn : Outport
  wires:
  TrueDurationTime9/1 -> Relational Operator/1
  Relational Operator/1 -> DSOther2Hi2Distractn/1
  Compare To Constant8/1 -> Logical Operator/5
  Compare To Constant4/1 -> Logical Operator/4
  Compare To Constant2/1 -> Logical Operator/3
  Compare To Constant/1 -> Logical Operator/1
  Compare To Constant1/1 -> Logical Operator/2
  canDistrctnQlty/1 -> Compare To Constant4/1, Compare To Constant8/1
  canDistrctnLevel/1 -> Compare To Constant2/1
  canHeadDetn/1 -> Compare To Constant1/1
  canDMSSts/1 -> Compare To Constant/1
  Logical Operator/1 -> TrueDurationTime9/1
  PtDSOther2Hi2Distractn/1 -> Relational Operator/2

== system PvtSubSys_DMS/Subsystem/DS/DriverStsConditnJudge/DSOther2Hi2DrowsnsJudge ==
  note: %Note
      | Conditions of drowsns state from other state to High2 as follow:
      | DMSSts_ACC is 0x02: Active
      | && HeadDetn is 0x01: Yes
      | && DrowsnsLevel_ACC is 0x3: Hi level Drowsiness
      | && DrowsnsQlty_ACC≥85%
      | && During time≥3s(adjustable)
  canDMSSts : Inport
  canHeadDetn : Inport  Port=2
  canDrowsnsLevel : Inport  Port=3
  PtDSOther2Hi2Drowsns : Inport  Port=4
  Compare To Constant : simulink/Logic and Bit Operations/Compare To Constant  relop===  const=2  OutDataTypeStr=boolean
  Compare To Constant1 : simulink/Logic and Bit Operations/Compare To Constant  relop===  const=1  OutDataTypeStr=boolean
  Compare To Constant2 : simulink/Logic and Bit Operations/Compare To Constant  relop===  const=3  OutDataTypeStr=boolean
  Logical Operator : Logic  Inputs=3  AllPortsSameDT=off  OutDataTypeStr=boolean
  Relational Operator : RelationalOperator  OutDataTypeStr=boolean  RndMeth=Simplest
  TrueDurationTime9 : TrueDurationTime/TrueDurationTime  TCycle=0.02
  DSOther2Hi2Drowsns : Outport
  wires:
  Logical Operator/1 -> TrueDurationTime9/1
  canDMSSts/1 -> Compare To Constant/1
  canHeadDetn/1 -> Compare To Constant1/1
  canDrowsnsLevel/1 -> Compare To Constant2/1
  Relational Operator/1 -> DSOther2Hi2Drowsns/1
  Compare To Constant1/1 -> Logical Operator/2
  Compare To Constant/1 -> Logical Operator/1
  Compare To Constant2/1 -> Logical Operator/3
  TrueDurationTime9/1 -> Relational Operator/1
  PtDSOther2Hi2Drowsns/1 -> Relational Operator/2
